simulink model "Part2_SimulinkModel"  (R2021a)
settings: Solver=VariableStepAuto  StartTime=0.0  StopTime=10.0  RelTol=1e-3  EnableMultiTasking=on
settings Model: Creator=Farhan  LastModifiedBy=david
settings SolverCC: AlgebraicLoopSolver=TrustRegion
settings DataIOCC: ReturnWorkspaceOutputs=off
settings OptimizationCC: LifeSpan=inf
settings DebuggingCC: SFUnexpectedBacktrackingDiag=warning  SFNoUnconditionalDefaultTransitionDiag=warning  SFMachineParentedDataDiag=warning  ArithmeticOperatorsInVariantConditions=warning
settings SFSimCC: SimUseLocalCustomCode=off  CustomCodeUndefinedFunction=UseInterfaceOnly
settings RTWCC: RTWUseLocalCustomCode=off
settings CodeAppCC: StateflowObjectComments=on
settings GRTTargetCC: TargetLangStandard=C89/C90 (ANSI)
settings ConfigComp: CovMetricSettings=dw  CovSaveCumulativeToWorkspaceVar=on  CovSaveSingleToWorkspaceVar=on  CovExternalEMLEnable=off

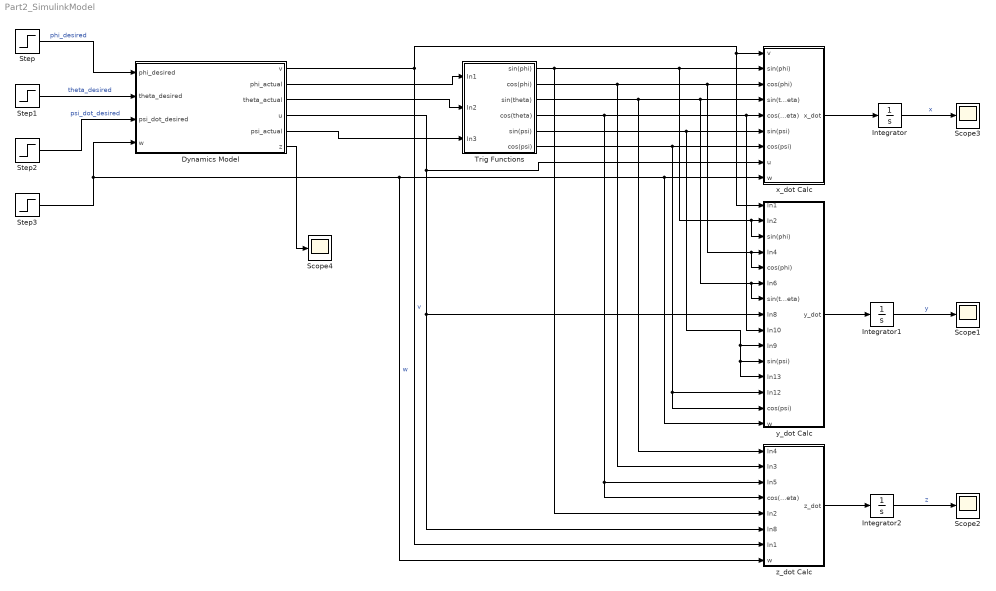
== system Part2_SimulinkModel ==
  Dynamics Model : Subsystem
  Integrator : Integrator
  Integrator1 : Integrator
  Integrator2 : Integrator
  Scope{1..4} (4 alike) : Scope
  Step{,1..3} (4 alike) : Step  SampleTime=0
  Trig Functions : Subsystem
  x_dot Calc : Subsystem
  y_dot Calc : Subsystem
  z_dot Calc : Subsystem
  wires:
  Step/1 -> Dynamics Model/1(phi_desired)  "phi_desired"
  Step1/1 -> Dynamics Model/2(theta_desired)  "theta_desired"
  Step2/1 -> Dynamics Model/3(psi_dot_desired)  "psi_dot_desired"
  Step3/1 -> z_dot Calc/8(w), y_dot Calc/15(w), x_dot Calc/9(w), Dynamics Model/4(w)  "w"
  Dynamics Model/2(phi_actual) -> Trig Functions/1(In1)
  Dynamics Model/3(theta_actual) -> Trig Functions/2(In2)
  Dynamics Model/5(psi_actual) -> Trig Functions/3(In3)
  Dynamics Model/1(v) -> z_dot Calc/7(In1), y_dot Calc/1(In1), x_dot Calc/1(v)  "v"
  Trig Functions/1(sin(phi)) -> z_dot Calc/5(In2), x_dot Calc/2(sin(phi)), y_dot Calc/3(sin(phi)), y_dot Calc/2(In2)
  Trig Functions/2(cos(phi)) -> z_dot Calc/2(In3), y_dot Calc/5(cos(phi)), y_dot Calc/4(In4), x_dot Calc/3(cos(phi))
  Trig Functions/3(sin(theta)) -> z_dot Calc/1(In4), y_dot Calc/7(sin(theta)), y_dot Calc/6(In6), x_dot Calc/4(sin(theta))
  Dynamics Model/4(u) -> z_dot Calc/6(In8), y_dot Calc/8(In8), x_dot Calc/8(u)
  Trig Functions/4(cos(theta)) -> y_dot Calc/9(In10), x_dot Calc/5(cos(theta)), z_dot Calc/4(cos(theta)), z_dot Calc/3(In5)
  Trig Functions/5(sin(psi)) -> y_dot Calc/12(In13), y_dot Calc/11(sin(psi)), y_dot Calc/10(In9), x_dot Calc/6(sin(psi))
  Trig Functions/6(cos(psi)) -> y_dot Calc/14(cos(psi)), y_dot Calc/13(In12), x_dot Calc/7(cos(psi))
  x_dot Calc/1(x_dot) -> Integrator/1
  Integrator/1 -> Scope3/1  "x"
  y_dot Calc/1(y_dot) -> Integrator1/1
  Integrator1/1 -> Scope1/1  "y"
  z_dot Calc/1(z_dot) -> Integrator2/1
  Integrator2/1 -> Scope2/1  "z"
  Dynamics Model/6(z) -> Scope4/1

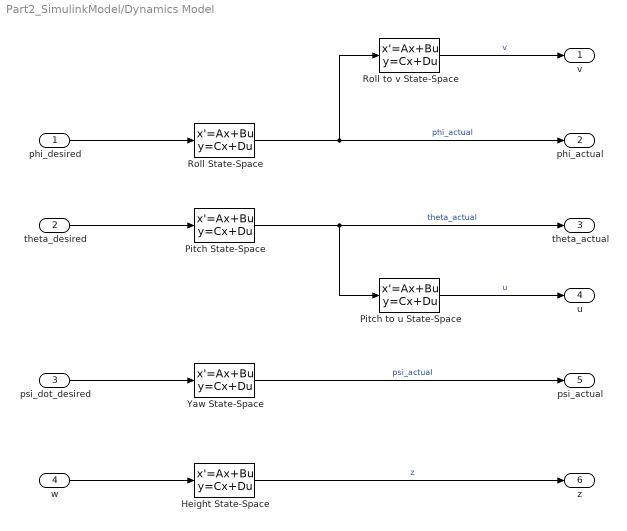
== system Part2_SimulinkModel/Dynamics Model ==
  phi_desired : Inport
  theta_desired : Inport  Port=2
  psi_dot_desired : Inport  Port=3
  w : Inport  Port=4
  Height State-Space : StateSpace  A=[-5.82 -3.6046*exp(1)^-6; 3.8147*exp(1)^-6 0]  B=[1024; 0]  C=[1.4907*exp(1)^-4 1.3191*exp(1)^3]  D=0  InitialCondition=0  ContinuousStateAttributes='Height'
  Pitch State-Space : StateSpace  A=[-3.9784 -2.9796; 4 0]  B=[2; 0]  C=[1.2569 0.6083]  D=0  InitialCondition=0  ContinuousStateAttributes='Pitch'
  Pitch to u State-Space : StateSpace  A=-0.665  B=2  C=-3.0772  D=0  InitialCondition=0  ContinuousStateAttributes='Pitch_to_u'
  Roll State-Space : StateSpace  A=[-4.2683 -3.1716; 4 0]  B=[2; 0]  C=[0.7417 0.4405]  D=0  InitialCondition=0  ContinuousStateAttributes='Roll'
  Roll to v State-Space : StateSpace  A=-0.4596  B=2  C=2.3868  D=0  InitialCondition=0  ContinuousStateAttributes='Roll_to_v'
  Yaw State-Space : StateSpace  A=-0.0059  C=1.2653  D=0  InitialCondition=0  ContinuousStateAttributes='Yaw'
  v : Outport
  phi_actual : Outport  Port=2
  theta_actual : Outport  Port=3
  u : Outport  Port=4
  psi_actual : Outport  Port=5
  z : Outport  Port=6
  wires:
  Yaw State-Space/1 -> psi_actual/1  "psi_actual"
  w/1 -> Height State-Space/1
  Height State-Space/1 -> z/1  "z"
  Roll State-Space/1 -> phi_actual/1, Roll to v State-Space/1  "phi_actual"
  theta_desired/1 -> Pitch State-Space/1
  psi_dot_desired/1 -> Yaw State-Space/1
  Pitch State-Space/1 -> theta_actual/1, Pitch to u State-Space/1  "theta_actual"
  phi_desired/1 -> Roll State-Space/1
  Roll to v State-Space/1 -> v/1  "v"
  Pitch to u State-Space/1 -> u/1  "u"

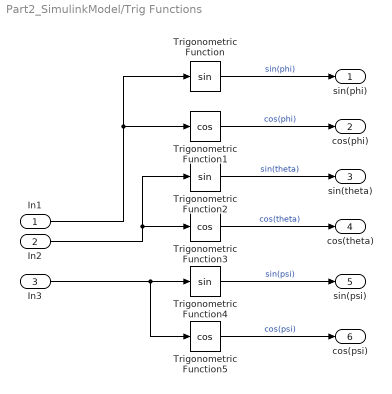
== system Part2_SimulinkModel/Trig Functions ==
  In1 : Inport
  In2 : Inport  Port=2
  In3 : Inport  Port=3
  Trigonometric Function : Trigonometry
  Trigonometric Function1 : Trigonometry  Operator=cos
  Trigonometric Function2 : Trigonometry
  Trigonometric Function3 : Trigonometry  Operator=cos
  Trigonometric Function4 : Trigonometry
  Trigonometric Function5 : Trigonometry  Operator=cos
  sin(phi) : Outport
  cos(phi) : Outport  Port=2
  sin(theta) : Outport  Port=3
  cos(theta) : Outport  Port=4
  sin(psi) : Outport  Port=5
  cos(psi) : Outport  Port=6
  wires:
  In1/1 -> Trigonometric Function1/1, Trigonometric Function/1
  Trigonometric Function2/1 -> sin(theta)/1  "sin(theta)"
  In2/1 -> Trigonometric Function3/1, Trigonometric Function2/1
  Trigonometric Function1/1 -> cos(phi)/1  "cos(phi)"
  In3/1 -> Trigonometric Function5/1, Trigonometric Function4/1
  Trigonometric Function4/1 -> sin(psi)/1  "sin(psi)"
  Trigonometric Function/1 -> sin(phi)/1  "sin(phi)"
  Trigonometric Function3/1 -> cos(theta)/1  "cos(theta)"
  Trigonometric Function5/1 -> cos(psi)/1  "cos(psi)"

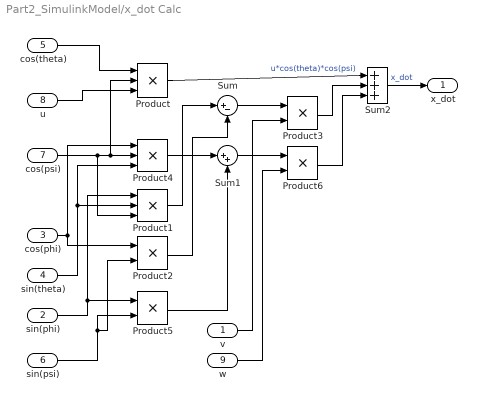
== system Part2_SimulinkModel/x_dot Calc ==
  v : Inport
  sin(phi) : Inport  Port=2
  cos(phi) : Inport  Port=3
  sin(theta) : Inport  Port=4
  cos(theta) : Inport  Port=5
  sin(psi) : Inport  Port=6
  cos(psi) : Inport  Port=7
  u : Inport  Port=8
  w : Inport  Port=9
  Product : Product  Inputs=3
  Product1 : Product  Inputs=3
  Product{2..3,5..6} (4 alike) : Product
  Product4 : Product  Inputs=3
  Sum : Sum  Inputs=|+-
  Sum1 : Sum  Inputs=|++
  Sum2 : Sum  Inputs=|+++
  x_dot : Outport
  wires:
  w/1 -> Product6/2
  Product5/1 -> Sum1/2
  Sum2/1 -> x_dot/1  "x_dot"
  Product/1 -> Sum2/1  "u*cos(theta)*cos(psi)"
  Product1/1 -> Sum/1
  sin(phi)/1 -> Product1/1, Product5/1
  v/1 -> Product3/2
  cos(psi)/1 -> Product/2, Product4/2, Product1/3
  Product2/1 -> Sum/2
  Sum/1 -> Product3/1
  Product3/1 -> Sum2/2
  cos(phi)/1 -> Product2/1, Product4/1
  cos(theta)/1 -> Product/1
  u/1 -> Product/3
  Sum1/1 -> Product6/1
  Product6/1 -> Sum2/3
  Product4/1 -> Sum1/1
  sin(psi)/1 -> Product5/2, Product2/2
  sin(theta)/1 -> Product4/3, Product1/2

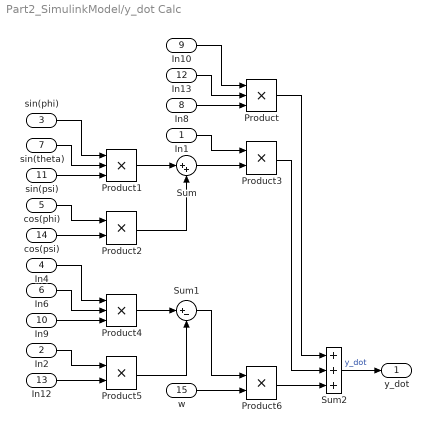
== system Part2_SimulinkModel/y_dot Calc ==
  In1 : Inport
  In2 : Inport  Port=2
  sin(phi) : Inport  Port=3
  In4 : Inport  Port=4
  cos(phi) : Inport  Port=5
  In6 : Inport  Port=6
  sin(theta) : Inport  Port=7
  In8 : Inport  Port=8
  In10 : Inport  Port=9
  In9 : Inport  Port=10
  sin(psi) : Inport  Port=11
  In13 : Inport  Port=12
  In12 : Inport  Port=13
  cos(psi) : Inport  Port=14
  w : Inport  Port=15
  Product : Product  Inputs=3
  Product1 : Product  Inputs=3
  Product{2..3,5..6} (4 alike) : Product
  Product4 : Product  Inputs=3
  Sum : Sum  Inputs=|++
  Sum1 : Sum  Inputs=|+-
  Sum2 : Sum  Inputs=+++
  y_dot : Outport
  wires:
  Sum/1 -> Product3/2
  Product5/1 -> Sum1/2
  sin(phi)/1 -> Product1/1
  In8/1 -> Product/3
  Product6/1 -> Sum2/3
  In6/1 -> Product4/2
  cos(phi)/1 -> Product2/1
  cos(psi)/1 -> Product2/2
  In1/1 -> Product3/1
  Product/1 -> Sum2/1
  Sum2/1 -> y_dot/1  "y_dot"
  In4/1 -> Product4/1
  Product4/1 -> Sum1/1
  Product2/1 -> Sum/2
  In9/1 -> Product4/3
  sin(theta)/1 -> Product1/2
  In13/1 -> Product/2
  Product3/1 -> Sum2/2
  w/1 -> Product6/2
  In10/1 -> Product/1
  sin(psi)/1 -> Product1/3
  In2/1 -> Product5/1
  Sum1/1 -> Product6/1
  Product1/1 -> Sum/1
  In12/1 -> Product5/2

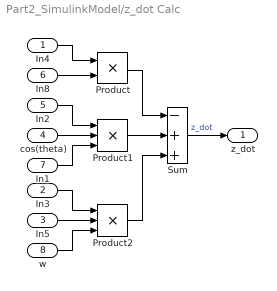
== system Part2_SimulinkModel/z_dot Calc ==
  In4 : Inport
  In3 : Inport  Port=2
  In5 : Inport  Port=3
  cos(theta) : Inport  Port=4
  In2 : Inport  Port=5
  In8 : Inport  Port=6
  In1 : Inport  Port=7
  w : Inport  Port=8
  Product : Product
  Product1 : Product  Inputs=3
  Product2 : Product  Inputs=3
  Sum : Sum  Inputs=-++
  z_dot : Outport
  wires:
  In4/1 -> Product/1
  In2/1 -> Product1/1
  w/1 -> Product2/3
  In1/1 -> Product1/3
  cos(theta)/1 -> Product1/2
  Product2/1 -> Sum/3
  In8/1 -> Product/2
  Product/1 -> Sum/1
  In3/1 -> Product2/1
  Sum/1 -> z_dot/1  "z_dot"
  In5/1 -> Product2/2
  Product1/1 -> Sum/2
